simulink model "AreaCoverageTestHarness"  (R2016a)
settings: Solver=FixedStepDiscrete  StartTime=0.0  StopTime=6000  FixedStep=0.005  RelTol=1e-3
values from neighbouring files (symbols this model uses):
  BLOCK_SIZE = CAL_BLOCK_SIZE    [AreaCoverageCalib.m]    (also in room_V1.m = 20; room_V3.m = 20)
  EAST = 0    [AreaCoverageCalib.m]
  ERRVAL = 5    [AreaCoverageCalib.m]
  initXSim = 35    [AreaCoverageCalib.m]
  initYSim = 50    [AreaCoverageCalib.m]
  MAX_SPEED = 1000    [AreaCoverageCalib.m]
  MOTOR_HIGH = CAL_MOTOR_HIGH    [AreaCoverageCalib.m]
  MOTOR_LOW = CAL_MOTOR_LOW    [AreaCoverageCalib.m]
  NORTH = 270    [AreaCoverageCalib.m]
  PLOT_SAMPLE = 10    [AreaCoverageCalib.m]
  ROB_LENG = CAL_ROBO_LENG    [AreaCoverageCalib.m]
  ROB_WHEEL_R = .15    (= 0.15)    [AreaCoverageCalib.m]
  room = uint8(ones(side_size , side_size)*255)    [room_V1.m]    (also in room_V3.m)
  ROOM_SIDE_SIZE = CAL_ROOM_SIDE_SIZE    [AreaCoverageCalib.m]    (also in room_V1.m = 20; room_V3.m = 20)
  SAMPLE_TIME = 0.001    [AreaCoverageCalib.m]
  SOUTH = 90    [AreaCoverageCalib.m]
  STEP_SIZE = 5    [AreaCoverageCalib.m]
  WEST = 180    [AreaCoverageCalib.m]
undefined symbols (not defined in the file or in its folder): ROBO_LENG, sigbuilder_block
libraries: simulink x4
(part 2 of 2)

== stateflow chart AreaCoverageTestHarness/Robot/RoomFilterSystem/Chart ==
  state hitFlag = westHitCheck(c_x, c_y) [function]
    (default) -> (junction 455) : {xCount = relSizeUnit;
        | yCount = 1;}
    (junction 455) -> (junction 452) [order 1] : [room[c_x - xCount][c_y - yCount] == 0]// fourth quadrant up left
    (junction 456) -> (junction 455) : {
        | xCount--;
        | yCount++;
        | }
    (junction 455) -> (junction 454) [order 2]
    (junction 452) -> (junction 451)
    (junction 454) -> (junction 456) [order 1] : [xCount > 0]
    (junction 454) -> (junction 450) [order 2] : {xCount = relSizeUnit;}
    (junction 450) -> (junction 451) [order 1] : [room[c_x - xCount][c_y] == 0]// West
    (junction 450) -> (junction 448) [order 2] : {xCount = relSizeUnit;
        | yCount = 1;}
    (junction 451) -> (junction 447)
    (junction 448) -> (junction 447) [order 1] : [room[c_x - xCount][c_y + yCount] == 0]// third quadrant down left
    (junction 446) -> (junction 448) : {
        | xCount--;
        | yCount++;
        | }
    (junction 448) -> (junction 453) [order 2]
    (junction 447) -> (junction 443) : {hitFlag = true;}
    (junction 453) -> (junction 446) [order 1] : [xCount > 0]
    (junction 453) -> (junction 445) [order 2] : {hitFlag = false;}
    (junction 443) -> (junction 445)
  state hitFlag = southHitCheck(c_x, c_y) [function]
    (default) -> (junction 387) : {
        | xCount = relSizeUnit;
        | yCount = 1;
        | }
    (junction 387) -> (junction 384) [order 1] : [room[c_x - xCount][c_y + yCount] == 0]// third quadrant down left
    (junction 388) -> (junction 387) : {
        | xCount--;
        | yCount++;
        | }
    (junction 387) -> (junction 386) [order 2]
    (junction 384) -> (junction 383)
    (junction 386) -> (junction 388) [order 1] : [xCount > 0]
    (junction 386) -> (junction 382) [order 2] : {yCount = relSizeUnit;}
    (junction 382) -> (junction 383) [order 1] : [room[c_x][c_y + yCount] == 0]// south
    (junction 382) -> (junction 380) [order 2] : {xCount = relSizeUnit;
        | yCount = 1;}
    (junction 383) -> (junction 379)
    (junction 380) -> (junction 379) [order 1] : [room[c_x + xCount][c_y + yCount] == 0]// second quadrant down right
    (junction 378) -> (junction 380) : {
        | xCount--;
        | yCount++;
        | }
    (junction 380) -> (junction 385) [order 2]
    (junction 379) -> (junction 375) : {hitFlag = true;}
    (junction 385) -> (junction 378) [order 1] : [xCount > 0]
    (junction 385) -> (junction 377) [order 2] : {hitFlag = false;}
    (junction 375) -> (junction 377)
  state hitFlag = eastHitCheck(c_x, c_y) [function]
    (default) -> (junction 421) : {xCount = relSizeUnit;
        | yCount = 1;}
    (junction 421) -> (junction 418) [order 1] : [room[c_x + xCount][c_y + yCount] == 0]// second quadrant down right
    (junction 422) -> (junction 421) : {
        | xCount--;
        | yCount++;
        | }
    (junction 421) -> (junction 420) [order 2]
    (junction 418) -> (junction 417)
    (junction 420) -> (junction 422) [order 1] : [xCount > 0]
    (junction 420) -> (junction 416) [order 2] : {xCount = relSizeUnit;}
    (junction 416) -> (junction 417) [order 1] : [room[c_x + xCount][c_y] == 0]// East
    (junction 416) -> (junction 414) [order 2] : {xCount = 1;
        | yCount = relSizeUnit;}
    (junction 417) -> (junction 413)
    (junction 414) -> (junction 413) [order 1] : [room[c_x + xCount][c_y - yCount] == 0]// first quadrant up right
    (junction 412) -> (junction 414) : {
        | xCount++;
        | yCount--;
        | }
    (junction 414) -> (junction 419) [order 2]
    (junction 413) -> (junction 409) : {hitFlag = true;}
    (junction 419) -> (junction 412) [order 1] : [yCount > 0]
    (junction 419) -> (junction 411) [order 2] : {hitFlag = false;}
    (junction 409) -> (junction 411)
  state hitFlag = northHitCheck(c_x, c_y) [function]
    (default) -> (junction 337) : {xCount = relSizeUnit;
        | yCount = 1;}
    (junction 337) -> (junction 335) [order 1] : [room[c_x - xCount][c_y - yCount] == 0]// fourth quadrant up left
    (junction 336) -> (junction 337) : {
        | xCount--;
        | yCount++;
        | }
    (junction 337) -> (junction 332) [order 2]
    (junction 335) -> (junction 345)
    (junction 332) -> (junction 336) [order 1] : [xCount > 0]
    (junction 332) -> (junction 344) [order 2] : {yCount = relSizeUnit;}
    (junction 344) -> (junction 345) [order 1] : [room[c_x][c_y - yCount] == 0]// north
    (junction 344) -> (junction 355) [order 2] : {xCount = 1;
        | yCount = relSizeUnit;}
    (junction 345) -> (junction 353)
    (junction 355) -> (junction 353) [order 1] : [room[c_x + xCount][c_y - yCount] == 0]// first quadrant up right
    (junction 354) -> (junction 355) : {
        | xCount++;
        | yCount--;
        | }
    (junction 355) -> (junction 350) [order 2]
    (junction 353) -> (junction 359) : {hitFlag = true;}
    (junction 350) -> (junction 354) [order 1] : [yCount > 0]
    (junction 350) -> (junction 360) [order 2] : {hitFlag = false;}
    (junction 359) -> (junction 360)
  state noHit
    entry:
    hit_BOOL = false;
  state HitCalcHeading
    entry:
    hit_BOOL = true;
    during:
    c_x = x_raw - 1;
    c_y = y_raw - 1;
    (default) -> (junction 163)
    (junction 163) -> (junction 164) [order 1] : [(theta <= 270+ERRVAL) && (theta >= 270 - ERRVAL)]//NORTH
    (junction 163) -> (junction 165) [order 2]
    (junction 164) -> (junction 178) : {heading = NORTH;}
    (junction 165) -> (junction 166) [order 1] : [(theta <= 90+ERRVAL) && (theta >= 90-ERRVAL)]//SOUTH
    (junction 165) -> (junction 167) [order 2]
    (junction 166) -> (junction 177) : {heading = SOUTH;}
    (junction 167) -> (junction 168) [order 1] : [(theta <= 0+ERRVAL) || (theta >= 360-ERRVAL)]//EAST
    (junction 167) -> (junction 169) [order 2]
    (junction 168) -> (junction 176) : {heading = EAST;}
    (junction 169) -> (junction 170) [order 1] : [(theta <= 180+ERRVAL) && (theta >= 180-ERRVAL)]//WEST
    (junction 169) -> (junction 171) [order 2] : {heading = NONE;}
    (junction 170) -> (junction 175) : {heading = WEST;}
    (junction 171) -> (junction 172) [order 2] : [Vr == Vl]
    (junction 172) -> (junction 174) : {wrongHeading_BOOL = true;}
    (junction 171) -> (junction 173) [order 1]
    (junction 174) -> (junction 173)
    (junction 175) -> (junction 174) : {wrongHeading_BOOL = false;}
    (junction 176) -> (junction 175)
    (junction 177) -> (junction 176)
    (junction 178) -> (junction 177)
    (junction 173) -> (junction 179)
  state CalcHeading
    entry:
    y_out = y_raw ;
    x_out = x_raw ;
    c_x = x_raw - 1; // X and Y in C arrays are flipped
    c_y = y_raw - 1;
    during:
    y_out = y_raw;
    x_out = x_raw ;
    c_x = x_raw - 1; // X and Y in C arrays are flipped
    c_y = y_raw - 1;
    (default) -> (junction 66)
    (junction 66) -> (junction 67) [order 1] : [(theta <= 270+ERRVAL) && (theta >= 270 - ERRVAL)]//NORTH
    (junction 66) -> (junction 68) [order 2]
    (junction 67) -> (junction 75) : {heading = NORTH;}
    (junction 68) -> (junction 69) [order 1] : [(theta <= 90+ERRVAL) && (theta >= 90-ERRVAL)]//SOUTH
    (junction 68) -> (junction 70) [order 2]
    (junction 69) -> (junction 74) : {heading = SOUTH;}
    (junction 70) -> (junction 71) [order 1] : [(theta <= 0+ERRVAL) || (theta >= 360-ERRVAL)]//EAST
    (junction 70) -> (junction 80) [order 2]
    (junction 71) -> (junction 73) : {heading = EAST;}
    (junction 80) -> (junction 79) [order 1] : [(theta <= 180+ERRVAL) && (theta >= 180-ERRVAL)]//WEST
    (junction 80) -> (junction 128) [order 2] : {heading = NONE;}
    (junction 79) -> (junction 77) : {heading = WEST;}
    (junction 128) -> (junction 125) [order 2] : [Vr == Vl]
    (junction 125) -> (junction 126) : {wrongHeading_BOOL = true;}
    (junction 128) -> (junction 72) [order 1]
    (junction 126) -> (junction 72)
    (junction 77) -> (junction 126) : {wrongHeading_BOOL = false;}
    (junction 73) -> (junction 77)
    (junction 74) -> (junction 73)
    (junction 75) -> (junction 74)
    (junction 72) -> (junction 76)
  (default) -> noHit
  (junction 157) -> (junction 147) [order 3] : [(heading == NORTH) ...
      | && ((c_y - 1) >= 0)...
      | &&((c_x) >= 0)]
  (junction 147) -> noHit : [room[c_x][c_y - 1] == 255]
  (junction 146) -> noHit : [room[c_x + 1][c_y] == 255]
  (junction 157) -> (junction 146) [order 2] : [(heading == EAST) ...
      | && ((c_x) <= 150 - 1)...
      | && ((c_y) >= 0)]
  (junction 92) -> HitCalcHeading : [northHitCheck(c_x, c_y)]
  (junction 109) -> (junction 92) [order 2] : [(heading == NORTH) ...
      | && ((c_y - 1) >= 0)...
      | &&((c_x) >= 0)]
  CalcHeading -> CalcHeading [order 3] : [hasChanged(theta)]
  HitCalcHeading -> (junction 157) [order 1] : [(Vr > 0) && (Vl > 0)]//FORWARD
  (junction 157) -> (junction 148) [order 4] : [(heading == SOUTH) ...
      | && ((c_y + 1) <= 150 - 1)...
      | && ((c_x) >= 0)]
  (junction 157) -> (junction 145) [order 1] : [(heading == WEST) ...
      | && ((c_x - 1) >= 0)...
      | && ((c_y) >= 0)]
  (junction 148) -> noHit : [room[c_x][c_y + 1] == 255]
  (junction 97) -> HitCalcHeading : [eastHitCheck(c_x, c_y)]
  (junction 109) -> (junction 97) [order 4] : [(heading == EAST) ...
      | && ((c_x) <= 150 - 1)...
      | && ((c_y) >= 0)]
  CalcHeading -> (junction 109) [order 1] : [(Vr > 0) && (Vl > 0)]//FORWARD
  (junction 109) -> (junction 100) [order 1] : [(heading == SOUTH) ...
      | && ((c_y + 1) <= 150 - 1)...
      | && ((c_x) >= 0)]
  (junction 109) -> (junction 103) [order 3] : [(heading == WEST) ...
      | && ((c_x - 1) >= 0)...
      | && ((c_y) >= 0)]
  (junction 145) -> noHit : [room[c_x - 1][c_y] == 255]
  (junction 100) -> HitCalcHeading : [southHitCheck(c_x, c_y)]
  HitCalcHeading -> noHit [order 4]
  (junction 103) -> HitCalcHeading : [westHitCheck(c_x, c_y)]
  (junction 135) -> noHit : [room[c_y + 1][c_x] == 255]
  (junction 160) -> (junction 135) [order 1] : [(heading == NORTH) ...
      | && ((c_y + 1) <= 150 - 1)...
      | && ((c_x) >= 0)]
  (junction 111) -> (junction 113) [order 1] : [(heading == NORTH) ...
      | && ((c_y + 1) <= 150 - 1)...
      | && ((c_x) >= 0)]
  (junction 113) -> HitCalcHeading : [room[c_y + 1][c_x] == 0]
  CalcHeading -> (junction 111) [order 2] : [(Vr < 0) && (Vl < 0)]//BACKWARD
  (junction 111) -> (junction 114) [order 2] : [(heading == EAST) ...
      | && ((c_x - 1) >= 0)...
      | && ((c_y) >= 0)]
  (junction 111) -> (junction 115) [order 3] : [(heading == SOUTH) ...
      | && ((c_y - 1) >= 0)...
      | && ((c_x) >=0)]
  (junction 111) -> (junction 116) [order 4] : [(heading == WEST) ...
      | && ((c_x + 1) <= (150-1))...
      | && ((c_y) >= 0)]
  (junction 114) -> HitCalcHeading : [room[c_y][c_x - 1] == 0]
  HitCalcHeading -> (junction 160) [order 2] : [(Vr < 0) && (Vl < 0)]//BACKWARD
  (junction 160) -> (junction 138) [order 2] : [(heading == EAST) ...
      | && ((c_x - 1) >= 0)...
      | && ((c_y) >= 0)]
  (junction 138) -> noHit : [room[c_y][c_x - 1] == 255]
  (junction 160) -> (junction 134) [order 3] : [(heading == SOUTH) ...
      | && ((c_y - 1) >= 0)...
      | && ((c_x) >=0)]
  (junction 160) -> (junction 136) [order 4] : [(heading == WEST) ...
      | && ((c_x + 1) <= (150-1))...
      | && ((c_y) >= 0)]
  noHit -> CalcHeading
  (junction 115) -> HitCalcHeading : [(room[c_y - 1][c_x] == 0)]
  (junction 134) -> noHit : [room[c_y - 1][c_x] == 255]
  (junction 116) -> HitCalcHeading : [room[c_y][c_x + 1] == 0]
  HitCalcHeading -> HitCalcHeading [order 3] : [hasChanged(theta)]
  (junction 136) -> noHit : [room[c_y][c_x + 1] == 255]
  data: c_x function_input double; c_y function_input double; hitFlag function_output boolean; i temporary int8; c_x function_input double; c_y function_input double; hitFlag function_output boolean; i temporary int8; c_x function_input double; c_y function_input double; hitFlag function_output boolean; i temporary int8; c_x function_input double; c_y function_input double; hitFlag function_output boolean; i temporary int8; x_raw input; y_raw input; room input size=[ROOM_SIDE_SIZE*BLOCK_SIZE/4 ROOM_SIDE_SIZE*BLOCK_SIZE/4]; y_out output int32; x_out output int32; y_temp local int32; x_temp local int32; hit_BOOL output boolean; theta input; ERRVAL input; NORTH input; SOUTH input; EAST input; WEST input; NONE input; heading local int16; Vr input; Vl input; wrongHeading_BOOL output boolean; c_x local double; c_y local double; relSizeUnit constant double =uint8(ROB_LENG/STEP_SIZE/2); xCount local double; yCount local double

== stateflow chart AreaCoverageTestHarness/Robot/RoomFilterSystem/StepCalc/Chart ==
  state inStep
    entry:
    temp = 0;
    state wait
    (default) -> wait
    (junction 7) -> wait : [oldPos < pos]/temp++;
    wait -> (junction 5) [order 1] : [hasChanged(pos)]
    (junction 5) -> wait : [oldPos > pos]/temp--;
    wait -> (junction 7) [order 2] : [hasChanged(pos)]
  state IncrementStep
    entry:
    step++;
  state Start
    entry:
    step = pos;
  state decrementStep
    step--;
  (default) -> Start
  Start -> inStep
  inStep -> IncrementStep [order 1] : [temp >= STEP_SIZE]
  IncrementStep -> inStep
  decrementStep -> inStep
  inStep -> decrementStep [order 2] : [temp <= -STEP_SIZE]
  data: pos input; oldPos input; step output int32; temp local int8; STEP_SIZE input int8

== stateflow chart AreaCoverageTestHarness/Robot/OrientationCalculator/VelocityCalculator/Chart2 ==
  (default) -> (junction 96)
  (junction 96) -> (junction 110) [order 1] : [(!LeftMotorPosPin_BOOL && !LeftMotorNegPin_BOOL && !RightMotorPosPin_BOOL && !RightMotorNegPin_BOOL)...
      | || (LeftMotorPosPin_BOOL && LeftMotorNegPin_BOOL && !RightMotorPosPin_BOOL && !RightMotorNegPin_BOOL)...
      | || (!LeftMotorPosPin_BOOL && !LeftMotorNegPin_BOOL && RightMotorPosPin_BOOL && RightMotorNegPin_BOOL)...
      | || (LeftMotorPosPin_BOOL && LeftMotorNegPin_BOOL && RightMotorPosPin_BOOL && RightMotorNegPin_BOOL)]
  (junction 110) -> (junction 118) : {Vr  = 0;
      | Vl = 0;}
  (junction 96) -> (junction 100) [order 2]
  (junction 100) -> (junction 97) [order 1] : [(!LeftMotorPosPin_BOOL && !LeftMotorNegPin_BOOL && RightMotorPosPin_BOOL && !RightMotorNegPin_BOOL)...
      | || (!LeftMotorPosPin_BOOL && LeftMotorNegPin_BOOL && RightMotorPosPin_BOOL && RightMotorNegPin_BOOL)...
      | || (LeftMotorPosPin_BOOL && LeftMotorNegPin_BOOL && RightMotorPosPin_BOOL && !RightMotorNegPin_BOOL)...
      | || (!LeftMotorPosPin_BOOL && LeftMotorNegPin_BOOL && !RightMotorPosPin_BOOL && !RightMotorNegPin_BOOL)]
  (junction 97) -> (junction 122) : {Vr = MAX_SPEED;
      | Vl = 0;}
  (junction 100) -> (junction 99) [order 2]
  (junction 99) -> (junction 98) [order 1] : [(!LeftMotorPosPin_BOOL && !LeftMotorNegPin_BOOL && !RightMotorPosPin_BOOL && RightMotorNegPin_BOOL)...
      | || (LeftMotorPosPin_BOOL && !LeftMotorNegPin_BOOL && !RightMotorPosPin_BOOL && !RightMotorNegPin_BOOL)...
      | || (LeftMotorPosPin_BOOL && !LeftMotorNegPin_BOOL && RightMotorPosPin_BOOL && RightMotorNegPin_BOOL)...
      | || (LeftMotorPosPin_BOOL && LeftMotorNegPin_BOOL && !RightMotorPosPin_BOOL && RightMotorNegPin_BOOL)]
  (junction 98) -> (junction 86) : {Vr = 0;
      | Vl = MAX_SPEED;}
  (junction 99) -> (junction 87) [order 2]
  (junction 87) -> (junction 101) [order 1] : [(!LeftMotorPosPin_BOOL && LeftMotorNegPin_BOOL && RightMotorPosPin_BOOL && !RightMotorNegPin_BOOL)]
  (junction 87) -> (junction 102) [order 2]
  (junction 101) -> (junction 130) : {Vr = MAX_SPEED;
      | Vl = -MAX_SPEED;}
  (junction 102) -> (junction 104) [order 1] : [(LeftMotorPosPin_BOOL && !LeftMotorNegPin_BOOL && !RightMotorPosPin_BOOL && RightMotorNegPin_BOOL)]
  (junction 102) -> (junction 133) [order 2]
  (junction 104) -> (junction 88) : {Vr = -MAX_SPEED;
      | Vl = MAX_SPEED;}
  (junction 133) -> (junction 105) [order 1] : [(LeftMotorPosPin_BOOL && !LeftMotorNegPin_BOOL && RightMotorPosPin_BOOL && !RightMotorNegPin_BOOL)]
  (junction 133) -> (junction 90) [order 2]
  (junction 105) -> (junction 89) : {Vr = MAX_SPEED;
      | Vl = MAX_SPEED;}
  (junction 90) -> (junction 94) [order 1] : [(!LeftMotorPosPin_BOOL && LeftMotorNegPin_BOOL && !RightMotorPosPin_BOOL && RightMotorNegPin_BOOL)]
  (junction 90) -> (junction 91) [order 2]
  (junction 94) -> (junction 127) : {Vr = -MAX_SPEED;
      | Vl = -MAX_SPEED;}
  (junction 127) -> (junction 91)
  (junction 89) -> (junction 127)
  (junction 88) -> (junction 89)
  (junction 130) -> (junction 88)
  (junction 86) -> (junction 130)
  (junction 122) -> (junction 86)
  (junction 118) -> (junction 122)
  (junction 91) -> (junction 119)
  data: LeftMotorPosPin_BOOL input; LeftMotorNegPin_BOOL input; RightMotorPosPin_BOOL input; RightMotorNegPin_BOOL input; Vr output int16 =0; Vl output int16 =0; MAX_SPEED input int16

== stateflow chart AreaCoverageTestHarness/Robot/RoomFilterSystem/StepCalc1/Chart ==
  state inStep
    entry:
    temp = 0;
    state wait
    (default) -> wait
    (junction 7) -> wait : [oldPos < pos]/temp++;
    wait -> (junction 5) [order 1] : [hasChanged(pos)]
    (junction 5) -> wait : [oldPos > pos]/temp--;
    wait -> (junction 7) [order 2] : [hasChanged(pos)]
  state IncrementStep
    entry:
    step++;
  state Start
    entry:
    step = pos;
  state decrementStep
    step--;
  (default) -> Start
  Start -> inStep
  inStep -> IncrementStep [order 1] : [temp >= STEP_SIZE]
  IncrementStep -> inStep
  decrementStep -> inStep
  inStep -> decrementStep [order 2] : [temp <= -STEP_SIZE]
  data: pos input; oldPos input; step output int32; temp local int8; STEP_SIZE input int8

== stateflow chart AreaCoverageTestHarness/Robot/ULS_Calc/ULS_Calculation ==
  state WestCalc
    entry:
    leftCounter = y - 1;
    rightCounter = y - 1;
    ULSL = 0;
    ULSR = 0;
    startLeft = true;
    startRight = true;
    state ULSL [parallel]
      settings: executionOrder=2
      (default) -> (junction 333)
      (junction 333) -> (junction 344) [order 1] : [leftCounter + 1 <= roomSize]
      (junction 336) -> (junction 333) : {ULSL++;}
      (junction 333) -> (junction 334) [order 2]
      (junction 344) -> (junction 335) : {leftCounter++;}
      (junction 334) -> (junction 336) [order 1] : [room[x-1][leftCounter] == 255]
      (junction 335) -> (junction 334)
      (junction 334) -> (junction 341) [order 2] : //if room[rightCounter][y - 1] == 0
    state ULSR [parallel]
      settings: executionOrder=1
      (default) -> (junction 347)
      (junction 347) -> (junction 358) [order 1] : [rightCounter - 1 >= 0]
      (junction 350) -> (junction 347) : {ULSR++;}
      (junction 347) -> (junction 348) [order 2]
      (junction 358) -> (junction 349) : {rightCounter--;}
      (junction 348) -> (junction 350) [order 1] : [room[x-1][rightCounter] == 255]
      (junction 349) -> (junction 348)
      (junction 348) -> (junction 355) [order 2] : //if room[rightCounter][y - 1] == 0
  state NorthCalc
    entry:
    leftCounter = x-1;
    rightCounter = x-1;
    ULSL = 0;
    ULSR = 0;
    startLeft = true;
    startRight = true;
    state ULSL [parallel]
      settings: executionOrder=1
      (default) -> (junction 232)
      (junction 232) -> (junction 236) [order 1] : [leftCounter - 1 >= 0]
      (junction 234) -> (junction 232) : {ULSL++;}
      (junction 232) -> (junction 193) [order 2]
      (junction 236) -> (junction 237) : {leftCounter--;}
      (junction 193) -> (junction 234) [order 1] : [room[leftCounter][y-1] == 255]
      (junction 237) -> (junction 193)
      (junction 193) -> (junction 233) [order 2]
    state ULSR [parallel]
      settings: executionOrder=2
      (default) -> (junction 258)
      (junction 258) -> (junction 250) [order 1] : [rightCounter + 1 <= roomSize]
      (junction 251) -> (junction 258) : {ULSR++;}
      (junction 258) -> (junction 253) [order 2]
      (junction 250) -> (junction 271) : {rightCounter++;}
      (junction 253) -> (junction 251) [order 1] : [room[rightCounter][y - 1] == 255]
      (junction 271) -> (junction 253)
      (junction 253) -> (junction 272) [order 2] : //if room[rightCounter][y - 1] == 0
  state CalcHeading
    (default) -> (junction 2)
    (junction 2) -> (junction 3) [order 1] : [(theta <= 270+ERRVAL) && (theta >= 270 - ERRVAL)]//NORTH
    (junction 2) -> (junction 4) [order 2]
    (junction 3) -> (junction 17) : {heading = NORTH;}
    (junction 4) -> (junction 5) [order 1] : [(theta <= 90+ERRVAL) && (theta >= 90-ERRVAL)]//SOUTH
    (junction 4) -> (junction 6) [order 2]
    (junction 5) -> (junction 16) : {heading = SOUTH;}
    (junction 6) -> (junction 7) [order 1] : [(theta <= 0+ERRVAL) || (theta >= 360-ERRVAL)]//EAST
    (junction 6) -> (junction 8) [order 2]
    (junction 7) -> (junction 15) : {heading = EAST;}
    (junction 8) -> (junction 9) [order 1] : [(theta <= 180+ERRVAL) && (theta >= 180-ERRVAL)]//WEST
    (junction 8) -> (junction 10) [order 2] : {heading = NONE;}
    (junction 9) -> (junction 14) : {heading = WEST;}
    (junction 10) -> (junction 11) [order 1] : [Vr == Vl]
    (junction 11) -> (junction 13) : {wrongHeading_BOOL = true;}
    (junction 10) -> (junction 12) [order 2]
    (junction 13) -> (junction 12)
    (junction 14) -> (junction 13) : {wrongHeading_BOOL = false;}
    (junction 15) -> (junction 14)
    (junction 16) -> (junction 15)
    (junction 17) -> (junction 16)
    (junction 12) -> (junction 18)
  state EastCalc
    entry:
    leftCounter = y-1;
    rightCounter = y-1;
    ULSL = 0;
    ULSR = 0;
    startLeft = true;
    startRight = true;
    state ULSL [parallel]
      settings: executionOrder=2
      (default) -> (junction 305)
      (junction 305) -> (junction 316) [order 1] : [leftCounter - 1 >= 0]
      (junction 308) -> (junction 305) : {ULSL++;}
      (junction 305) -> (junction 306) [order 2]
      (junction 316) -> (junction 307) : {leftCounter--;}
      (junction 306) -> (junction 308) [order 1] : [room[x-1][leftCounter] == 255]
      (junction 307) -> (junction 306)
      (junction 306) -> (junction 313) [order 2] : //if room[rightCounter][y - 1] == 0
    state ULSR [parallel]
      settings: executionOrder=1
      (default) -> (junction 319)
      (junction 319) -> (junction 330) [order 1] : [rightCounter + 1 <= roomSize]
      (junction 322) -> (junction 319) : {ULSR++;}
      (junction 319) -> (junction 320) [order 2]
      (junction 330) -> (junction 321) : {rightCounter++;}
      (junction 320) -> (junction 322) [order 1] : [room[x-1][rightCounter] == 255]
      (junction 321) -> (junction 320)
      (junction 320) -> (junction 327) [order 2] : //if room[rightCounter][y - 1] == 0
  state SouthCalc
    entry:
    leftCounter = x-1;
    rightCounter = x-1;
    ULSL = 0;
    ULSR = 0;
    startLeft = true;
    startRight = true;
    state ULSL [parallel]
      settings: executionOrder=1
      (default) -> (junction 278)
      (junction 278) -> (junction 288) [order 1] : [leftCounter + 1 <= roomSize]
      (junction 279) -> (junction 278) : {ULSL++;}
      (junction 278) -> (junction 286) [order 2]
      (junction 288) -> (junction 281) : {leftCounter++;}
      (junction 286) -> (junction 279) [order 1] : [room[leftCounter][y-1] == 255]
      (junction 281) -> (junction 286)
      (junction 286) -> (junction 283) [order 2] : //if room[leftCounter][y - 1] == 0
    state ULSR [parallel]
      settings: executionOrder=2
      (default) -> (junction 292)
      (junction 292) -> (junction 302) [order 1] : [rightCounter - 1 >= 0]
      (junction 293) -> (junction 292) : {ULSR++;}
      (junction 292) -> (junction 300) [order 2]
      (junction 302) -> (junction 295) : {rightCounter--;}
      (junction 300) -> (junction 293) [order 1] : [room[rightCounter][y - 1] == 255]
      (junction 295) -> (junction 300)
      (junction 300) -> (junction 297) [order 2] : //if room[rightCounter][y - 1] == 0
  (default) -> CalcHeading
  CalcHeading -> WestCalc [order 1] : [(heading == WEST) ...
      | && (hasChanged(heading)...
      | || hasChanged(x))]
      | /readingReady = false;
  CalcHeading -> NorthCalc [order 4] : [(heading == NORTH) ...
      | && (hasChanged(heading)...
      | || hasChanged(y))]
      | /readingReady = false;
  (junction 154) -> CalcHeading : [(room[x-1][rightCounter] == 0)...
      |  &&(room[x-1][leftCounter] == 0)]
      | /readingReady = true;
  WestCalc -> (junction 154) : [x-1 >= 0]
  EastCalc -> (junction 154) : [x-1 >= 0]
  NorthCalc -> (junction 117) : [y-1 >= 0]
  (junction 117) -> CalcHeading : [(room[rightCounter][y-1] == 0)...
      |  &&(room[leftCounter][y-1] == 0)]
      | /readingReady = true;
  SouthCalc -> (junction 117) : [y-1 >= 0]
  CalcHeading -> EastCalc [order 2] : [(heading == EAST) ...
      | && (hasChanged(heading)...
      | || hasChanged(x))]
      | /readingReady = false;
  CalcHeading -> SouthCalc [order 3] : [(heading == SOUTH) ...
      | && (hasChanged(heading)...
      | || hasChanged(y))]
      | /readingReady = false;
  CalcHeading -> CalcHeading [order 5] : [hasChanged(theta)]
  data: ERRVAL input; NORTH input; SOUTH input; EAST input; WEST input; NONE input; room input size=[ROOM_SIDE_SIZE*BLOCK_SIZE/4 ROOM_SIDE_SIZE*BLOCK_SIZE/4]; heading local int16; theta input; Vl input; Vr input; roomSize input; x input; y input; wrongHeading_BOOL output double; ULSL output double; ULSR output double; leftCounter local double; rightCounter local double; startLeft local boolean; startRight local boolean; readingReady output boolean

== matlab function AreaCoverageTestHarness/Robot/DetailedMap/MATLAB Function ==
  data: room input; X input; Y input; Theta input; ROOM_SIDE_SIZE parameter; clock input; BLOCK_SIZE parameter
function PlotterFunc(room, X, Y, Theta, ROOM_SIDE_SIZE, clock, BLOCK_SIZE)

persistent init;
persistent fig;

if isempty(fig)
    fig = figure;
end

if isempty(init)
    init = 0;
    %room = uint8(room');
    hold off;
    clf
    empty = 255;
    busy = 0;
    hold on
    offset = 0;
    for i = 1:length(room(1, :))
        for j = 1:length(room(:, 1))
            if room(i, j) == empty
%                 plot(i - offset, j - offset, '*b');
            else if room(i,j) == busy
                    plot(i - offset, j - offset, '.r');
                else 
                    plot(i - offset, j - offset, 'x');
                end
            end
        end
    end
    axis ij
end


delta = clock - init;
if(delta) >= 0.5
%     figure(fig);
    init = clock;
    Xplot = double(X);
    Yplot = double(Y);
        if clock
%             hold on
            lineLength = double(BLOCK_SIZE*0.25);
            opleft = double(sind(Theta+90) * (lineLength/2));
            adjleft = double(cosd(Theta+90) * (lineLength/2));
            yend = double(Yplot) + opleft;
            xend = double(Xplot) + adjleft;
            start = [double(Xplot) xend];
            finish = [double(Yplot) yend];

            opright = double(sind(Theta-90) * (lineLength/2));
            adjright = double(cosd(Theta-90) * (lineLength/2));

            plot(double(Xplot), double(Yplot), 'r*', 'MarkerSize', 10);
            hold on

            plot(start, finish, 'g', 'LineWidth', 3)
            plot(xend, yend, 'bx')
            yend = double(Yplot) + opright;
            xend = double(Xplot) + adjright;
            start = [double(Xplot) xend];
            finish = [double(Yplot) yend];
            plot(start, finish, 'g','LineWidth', 3)
            plot(xend, yend, 'bx')
%             hold off
%             xlim([-1*((ROOM_SIDE_SIZE * BLOCK_SIZE)/2) - 50 (ROOM_SIDE_SIZE * BLOCK_SIZE)/2 + 50]);
%             ylim([-1*((ROOM_SIDE_SIZE * BLOCK_SIZE)/2) - 50 (ROOM_SIDE_SIZE * BLOCK_SIZE)/2 + 50]);
            xlim([0 100]);
            ylim([0 100]);
            grid on
            grid minor
%                 hold off;

    %         axis ij
        end
end

== stateflow chart AreaCoverageTestHarness/Robot/PlotSampler ==
  (default) -> (junction 1)
  (junction 1) -> (junction 3) : {counter = counter + 1;...
      | Event_BOOL = false;}
  (junction 3) -> (junction 5) [order 1] : [counter >= PLOT_SAMPLE]
  (junction 3) -> (junction 9) [order 2] : /{Event_BOOL = false;}
  (junction 5) -> (junction 7) : {counter = 0;...
      | Event_BOOL = true;}
  (junction 7) -> (junction 9)
  data: counter local uint8; Event_BOOL output boolean; PLOT_SAMPLE input

== matlab function AreaCoverageTestHarness/Robot/DetailedMap/createMap/RoomV3/Room_V3 ==
  data: roomOut output size=[ROOM_SIDE_SIZE*BLOCK_SIZE/4 ROOM_SIDE_SIZE*BLOCK_SIZE/4] [0..255]; ROOM_SIDE_SIZE parameter; BLOCK_SIZE parameter
function roomOut = fcn(ROOM_SIDE_SIZE, BLOCK_SIZE)

persistent flag;
persistent room;
   side_size = ROOM_SIDE_SIZE * (BLOCK_SIZE/4);

if isempty(flag)
    flag = false;
    room = uint8(ones(side_size , side_size)*255);
end

if flag == false
   flag = true;
%     room = uint8(ones(ROOM_SIDE_SIZE , ROOM_SIDE_SIZE)*255);

    %% Draw room Boarders
    for rowNum = 1:(side_size)
        for colNum = 1: side_size
            if (rowNum <= BLOCK_SIZE/4) || (rowNum >= (side_size - BLOCK_SIZE/4))...
                    || (colNum <= BLOCK_SIZE/4) || (colNum >= side_size - BLOCK_SIZE/4)
    %                 || (rowNum == 2) || (rowNum == roomSize - 1)...
    %                 || (colNum == 2) || (colNum == roomSize-1)
                room(rowNum, colNum) = 0;
            end
        end
    end

    %% Draw room Obsticals
    scale = 5;
    %% insert Table
    room((9*scale - scale/2) + 0.5:(11*scale + scale/2) + 0.5, (7*scale - scale/4) + 0.5:(13*scale + scale/4 )+ 0.5) = 0;
 
    %% insert chairs
    room((17*scale - scale/2) + 0.5:(19*scale + scale/2) + 0.5, (5*scale - (scale)/2) + 0.5:(8*scale + (scale)/2 )+ 0.5) = 0;

%     room((15.5*scale - scale/2) + 0.5:(17.5*scale + scale/2) + 0.5, (13*scale - (scale)/2) + 0.5:(16*scale + (scale)/2 )+ 0.5) = 0;

    room((9*scale - scale/2) + 0.5:(12*scale + scale/2) + 0.5, (17*scale - (scale)/2) + 0.5:(19*scale + (scale)/2 )+ 0.5) = 0;
    
    x = (14:0.1:16.5);
    y = (16:0.1:19);
    depth = 5;
    for j = 1:depth*scale
        for i = 1:length(x)
            room(uint8((x(i)*scale - scale/2) + 0.5), uint8((y(i)*scale - scale/2) + 0.5)) = 0;
        end
        x = x + 0.1;
        y = y - 0.1;
    end
    
    
    x = (2:0.1:5);
    y = (16.5:0.1:19.5);
    depth = 5;
    for j = 1:depth*scale
        for i = 1:length(x)
            room(uint8((x(i)*scale - scale/2) + 0.5), uint8((y(i)*scale - scale/2) + 0.5)) = 0;
        end
        x = x + 0.1;
        y = y - 0.1;
    end
    
    room((2*scale - scale/2) + 0.5:(4*scale + scale/2) + 0.5, (6*scale - (scale)/2) + 0.5:(13*scale + (scale)/2 )+ 0.5) = 0;
  
    roomOut = room;
else
    roomOut = room;
end

== stateflow chart AreaCoverageTestHarness/Robot/EncoderTicksGenerator/SquareWaveCreatorLeft ==
  state BulbOn
    state Off
      entry:
      counter = 0;
      encoderTicks_BOOL = false;
      du:
      counter++;
    state On
      entry:
      counter = 0;
      encoderTicks_BOOL = true;
      du:
      counter++;
    (default) -> Off
    On -> Off : [counter >= (spdGain)]/counter = 0;
    Off -> On : [counter >= (spdGain)]/counter = 0;
  state BulbOff
    entry:
    encoderTicks_BOOL = 0;
  (default) -> BulbOff
  BulbOff -> BulbOn : [ControlSignal_BOOL_in]
  BulbOn -> BulbOff : [!ControlSignal_BOOL_in]
  data: ControlSignal_BOOL_in input; encoderTicks_BOOL output boolean; counter local uint16; spdGain input

== matlab function AreaCoverageTestHarness/Robot/GridMap/MATLAB Function ==
  data: room input; X input; Y input; Theta input; ROOM_SIDE_SIZE parameter; clock input; BLOCK_SIZE parameter
function PlotterFunc(room, X, Y, Theta, ROOM_SIDE_SIZE, clock, BLOCK_SIZE)

persistent init;
persistent fig1;

if isempty(fig1)
    fig1 = figure;
end

if isempty(init)
    init = 0;
    %room = uint8(room');
    hold off;
    clf
    empty = 255;
    busy = 0;
    hold on
    offset = 0;
    for i = 1:length(room(1, :))
        for j = 1:length(room(:, 1))
            if room(i, j) == empty
                plot(i - offset, j - offset, '*b');
            else if room(i,j) == busy
                    plot(i - offset, j - offset, 'or');
                else 
                    plot(i - offset, j - offset, 'x');
                end
            end
        end
    end
    axis ij
end

delta = clock - init;
if(delta) >= 0.5
    figure(fig1);
    init = clock;
%     X = X - 1;
%     Y = Y - 1;
        if clock
            lineLength = double(BLOCK_SIZE*0.05);
            opleft = double(sind(Theta+90) * (lineLength/2));
            adjleft = double(cosd(Theta+90) * (lineLength/2));
            yend = double(Y) + opleft;
            xend = double(X) + adjleft;
            start = [double(X) xend];
            finish = [double(Y) yend];

            opright = double(sind(Theta-90) * (lineLength/2));
            adjright = double(cosd(Theta-90) * (lineLength/2));

            plot(double(X), double(Y), '*', 'MarkerSize', 10);
            hold on
            plot(start, finish, 'LineWidth', 3)
            plot(xend, yend, 'x')
            yend = double(Y) + opright;
            xend = double(X) + adjright;
            start = [double(X) xend];
            finish = [double(Y) yend];
            plot(start, finish, 'LineWidth', 3)
            plot(xend, yend, 'x')
%             hold off
            xlim([0 (ROOM_SIDE_SIZE)]);
            ylim([0 (ROOM_SIDE_SIZE)]);
            grid on
            grid minor
    %         axis ij
        end
end

== matlab function AreaCoverageTestHarness/Robot/createMap/MATLAB Function ==
  data: roomOut output size=[ROOM_SIDE_SIZE ROOM_SIDE_SIZE] [0..255]; ROOM_SIDE_SIZE parameter
function roomOut = fcn(  ROOM_SIDE_SIZE)

%persistent flag;
    room = uint8(ones(ROOM_SIDE_SIZE , ROOM_SIDE_SIZE)*255);
%if isempty(flag)
 %   flag = true;
%     room = uint8(ones(ROOM_SIDE_SIZE , ROOM_SIDE_SIZE)*255);

    %% Draw room Boarders
    for rowNum = 1:(ROOM_SIDE_SIZE)
        for colNum = 1: ROOM_SIDE_SIZE
            if (rowNum == 1) || (rowNum == ROOM_SIDE_SIZE)...
                    || (colNum == 1) || (colNum == ROOM_SIDE_SIZE)
    %                 || (rowNum == 2) || (rowNum == roomSize - 1)...
    %                 || (colNum == 2) || (colNum == roomSize-1)
                room(rowNum, colNum) = 0;
            end
        end
    end

    %% Draw room Obsticals

    %% insert Table
    room(4, 9) = 0;
    room(6, 9) = 0;
    room(4, 11) = 0;
    room(6, 11) = 0;

    %% insert box
    room(3:4, 4:5) = 0;

    %% insert soffa
    room(12:14, 8:13) = 0;

    %% insert LeglessTable
    room(7:11, 1:4) = 0;
    roomOut = room;
%else
  %  roomOut = room;
%end

== stateflow chart AreaCoverageTestHarness/Robot/ULS_Calc/ULS_Calculation1 ==
  state WestCalc
    entry:
    leftCounter = y - 1;
    rightCounter = y - 1;
    ULSL = 0;
    ULSR = 0;
    startLeft = true;
    startRight = true;
    state ULSL [parallel]
      settings: executionOrder=2
      (history)
      state ULSL_Calc
      state Hit
      WestCalc.ULSL.ULSL_Calc -> (junction 148) : [leftCounter + 1 <= roomSize]{leftCounter++;}
      (default) -> WestCalc.ULSL.ULSL_Calc
      (junction 148) -> WestCalc.ULSL.Hit [order 1] : [room[x-1][leftCounter] == 0]
          | /startLeft = false;
      (junction 148) -> WestCalc.ULSL.ULSL_Calc [order 2] : [room[x-1][leftCounter] == 255]
          | /ULSL++;
      WestCalc.ULSL.Hit -> WestCalc.ULSL.ULSL_Calc : [startLeft]
    state ULSR [parallel]
      settings: executionOrder=1
      (history)
      state ULSR_Calc1
      state Hit
      WestCalc.ULSR.ULSR_Calc1 -> (junction 147) : [rightCounter - 1 >= 0]{rightCounter--;}
      (default) -> WestCalc.ULSR.ULSR_Calc1
      (junction 147) -> WestCalc.ULSR.Hit [order 1] : [room[x-1][rightCounter] == 0]
          | /startRight = false;
      (junction 147) -> WestCalc.ULSR.ULSR_Calc1 [order 2] : [room[x-1][rightCounter] == 255]
          | /ULSR++;
      WestCalc.ULSR.Hit -> WestCalc.ULSR.ULSR_Calc1 : [startRight]
  state NorthCalc
    entry:
    leftCounter = x-1;
    rightCounter = x-1;
    ULSL = 0;
    ULSR = 0;
    startLeft = true;
    startRight = true;
    state ULSL [parallel]
      settings: executionOrder=2
      (history)
      state ULSL_Calc
      state Hit
      NorthCalc.ULSL.ULSL_Calc -> (junction 193) : [leftCounter - 1 >= 0]{leftCounter--;}
      (default) -> NorthCalc.ULSL.ULSL_Calc
      (junction 193) -> NorthCalc.ULSL.Hit [order 1] : [room[leftCounter][y-1]== 0]
          | /startLeft = false;
      (junction 193) -> NorthCalc.ULSL.ULSL_Calc [order 2] : [room[leftCounter][y-1] == 255]
          | /ULSL++;
      NorthCalc.ULSL.Hit -> NorthCalc.ULSL.ULSL_Calc : [startLeft]
    state ULSR [parallel]
      settings: executionOrder=1
      (history)
      state ULSR_Calc
      state Hit
      NorthCalc.ULSR.ULSR_Calc -> (junction 206) : [rightCounter + 1 <= roomSize]{rightCounter++;}
      (default) -> NorthCalc.ULSR.ULSR_Calc
      (junction 206) -> NorthCalc.ULSR.Hit [order 1] : [room[rightCounter][y - 1] == 0]
          | /startRight = false;
      (junction 206) -> NorthCalc.ULSR.ULSR_Calc [order 2] : [room[rightCounter][y - 1] == 255]
          | /ULSR++;
      NorthCalc.ULSR.Hit -> NorthCalc.ULSR.ULSR_Calc : [startRight]
  state CalcHeading
    (default) -> (junction 2)
    (junction 2) -> (junction 3) [order 1] : [(theta <= 270+ERRVAL) && (theta >= 270 - ERRVAL)]//NORTH
    (junction 2) -> (junction 4) [order 2]
    (junction 3) -> (junction 17) : {heading = NORTH;}
    (junction 4) -> (junction 5) [order 1] : [(theta <= 90+ERRVAL) && (theta >= 90-ERRVAL)]//SOUTH
    (junction 4) -> (junction 6) [order 2]
    (junction 5) -> (junction 16) : {heading = SOUTH;}
    (junction 6) -> (junction 7) [order 1] : [(theta <= 0+ERRVAL) || (theta >= 360-ERRVAL)]//EAST
    (junction 6) -> (junction 8) [order 2]
    (junction 7) -> (junction 15) : {heading = EAST;}
    (junction 8) -> (junction 9) [order 1] : [(theta <= 180+ERRVAL) && (theta >= 180-ERRVAL)]//WEST
    (junction 8) -> (junction 10) [order 2] : {heading = NONE;}
    (junction 9) -> (junction 14) : {heading = WEST;}
    (junction 10) -> (junction 11) [order 2] : [Vr == Vl]
    (junction 11) -> (junction 13) : {wrongHeading_BOOL = true;}
    (junction 10) -> (junction 12) [order 1]
    (junction 13) -> (junction 12)
    (junction 14) -> (junction 13) : {wrongHeading_BOOL = false;}
    (junction 15) -> (junction 14)
    (junction 16) -> (junction 15)
    (junction 17) -> (junction 16)
    (junction 12) -> (junction 18)
  state EastCalc
    entry:
    leftCounter = y-1;
    rightCounter = y-1;
    ULSL = 0;
    ULSR = 0;
    startLeft = true;
    startRight = true;
    state ULSL [parallel]
      settings: executionOrder=2
      (history)
      state ULSL_Calc
      state Hit
      EastCalc.ULSL.ULSL_Calc -> (junction 172) : [leftCounter - 1 >= 0]{leftCounter--;}
      (default) -> EastCalc.ULSL.ULSL_Calc
      (junction 172) -> EastCalc.ULSL.Hit [order 1] : [room[x-1][leftCounter] == 0]
          | /startLeft = false;
      (junction 172) -> EastCalc.ULSL.ULSL_Calc [order 2] : [room[x-1][leftCounter] == 255]
          | /ULSL++;
      EastCalc.ULSL.Hit -> EastCalc.ULSL.ULSL_Calc : [startLeft]
    state ULSR [parallel]
      settings: executionOrder=1
      (history)
      state ULSR_Calc1
      state Hit
      EastCalc.ULSR.ULSR_Calc1 -> (junction 185) : [rightCounter + 1 <= roomSize]{rightCounter++;}
      (default) -> EastCalc.ULSR.ULSR_Calc1
      (junction 185) -> EastCalc.ULSR.Hit [order 1] : [room[x-1][rightCounter] == 0]
          | /startRight = false;
      (junction 185) -> EastCalc.ULSR.ULSR_Calc1 [order 2] : [room[x-1][rightCounter] == 255]
          | /ULSR++;
      EastCalc.ULSR.Hit -> EastCalc.ULSR.ULSR_Calc1 : [startRight]
  state SouthCalc
    entry:
    leftCounter = x-1;
    rightCounter = x-1;
    ULSL = 0;
    ULSR = 0;
    startLeft = true;
    startRight = true;
    state ULSL [parallel]
      settings: executionOrder=2
      (history)
      state ULSL_Calc
      state Hit
      SouthCalc.ULSL.ULSL_Calc -> (junction 226) : [leftCounter + 1 <= roomSize]{leftCounter++;}
      (default) -> SouthCalc.ULSL.ULSL_Calc
      (junction 226) -> SouthCalc.ULSL.Hit [order 1] : [room[leftCounter][y-1] == 0]
          | /startLeft = false;
      (junction 226) -> SouthCalc.ULSL.ULSL_Calc [order 2] : [room[leftCounter][y-1] == 255]
          | /ULSL++;
      SouthCalc.ULSL.Hit -> SouthCalc.ULSL.ULSL_Calc : [startLeft]
    state ULSR [parallel]
      settings: executionOrder=1
      (history)
      state ULSR_Calc
      state Hit
      SouthCalc.ULSR.ULSR_Calc -> (junction 213) : [rightCounter - 1 >= 0]{rightCounter--;}
      (default) -> SouthCalc.ULSR.ULSR_Calc
      (junction 213) -> SouthCalc.ULSR.Hit [order 1] : [room[rightCounter][y - 1] == 0]
          | /startRight = false;
      (junction 213) -> SouthCalc.ULSR.ULSR_Calc [order 2] : [room[rightCounter][y - 1] == 255]
          | /ULSR++;
      SouthCalc.ULSR.Hit -> SouthCalc.ULSR.ULSR_Calc : [startRight]
  (default) -> CalcHeading
  CalcHeading -> WestCalc [order 1] : [(heading == WEST) ...
      | && (hasChanged(heading)...
      | || hasChanged(x))]
      | /readingReady = false;
  CalcHeading -> NorthCalc [order 4] : [(heading == NORTH) ...
      | && (hasChanged(heading)...
      | || hasChanged(y))]
      | /readingReady = false;
  WestCalc -> (junction 154) : [x-1 >= 0]
  (junction 154) -> CalcHeading : [(room[x-1][rightCounter] == 0)...
      |  &&(room[x-1][leftCounter] == 0)]
      | /readingReady = true;
  NorthCalc -> (junction 117) : [y-1 >= 0]
  EastCalc -> (junction 154) : [x-1 >= 0]
  (junction 117) -> CalcHeading : [(room[rightCounter][y-1] == 0)...
      |  &&(room[leftCounter][y-1] == 0)]
      | /readingReady = true;
  SouthCalc -> (junction 117) : [y-1 >= 0]
  CalcHeading -> EastCalc [order 2] : [(heading == EAST) ...
      | && (hasChanged(heading)...
      | || hasChanged(x))]
      | /readingReady = false;
  CalcHeading -> SouthCalc [order 3] : [(heading == SOUTH) ...
      | && (hasChanged(heading)...
      | || hasChanged(y))]
      | /readingReady = false;
  CalcHeading -> CalcHeading [order 5] : [hasChanged(theta)]
  data: ERRVAL input; NORTH input; SOUTH input; EAST input; WEST input; NONE input; room input size=[ROOM_SIDE_SIZE*BLOCK_SIZE/4 ROOM_SIDE_SIZE*BLOCK_SIZE/4]; heading local int16; theta input; Vl input; Vr input; roomSize input; x input; y input; wrongHeading_BOOL output double; ULSL output double; ULSR output double; leftCounter local double; rightCounter local double; startLeft local boolean; startRight local boolean; readingReady output boolean

== matlab function AreaCoverageTestHarness/Robot/DetailedMap/createMap/RoomV1/Room_V1 ==
  data: roomOut output size=[ROOM_SIDE_SIZE*BLOCK_SIZE/4 ROOM_SIDE_SIZE*BLOCK_SIZE/4] [0..255]; ROOM_SIDE_SIZE parameter; BLOCK_SIZE parameter
function roomOut = fcn(ROOM_SIDE_SIZE, BLOCK_SIZE)

persistent flag;
persistent room;
   side_size = ROOM_SIDE_SIZE * (BLOCK_SIZE/4);

if isempty(flag)
    flag = false;
    room = uint8(ones(side_size , side_size)*255);
end

if flag == false
   flag = true;
%     room = uint8(ones(ROOM_SIDE_SIZE , ROOM_SIDE_SIZE)*255);

    %% Draw room Boarders
    for rowNum = 1:(side_size)
        for colNum = 1: side_size
            if (rowNum <= BLOCK_SIZE/4) || (rowNum >= (side_size - BLOCK_SIZE/4))...
                    || (colNum <= BLOCK_SIZE/4) || (colNum >= side_size - BLOCK_SIZE/4)
    %                 || (rowNum == 2) || (rowNum == roomSize - 1)...
    %                 || (colNum == 2) || (colNum == roomSize-1)
                room(rowNum, colNum) = 0;
            end
        end
    end

    %% Draw room Obsticals
    scale = 5;
    %% insert Table
    room((4*scale - scale/2) + 0.5:(4*scale + scale/2) + 0.5, (9*scale - scale/2) + 0.5:(9*scale + scale/2 )+ 0.5) = 0;
    room((6*scale - scale/2) + 0.5:(6*scale + scale/2) + 0.5, (9*scale - scale/2) + 0.5:(9*scale + scale/2 )+ 0.5) = 0;
    room((4*scale - scale/2) + 0.5:(4*scale + scale/2) + 0.5, (11*scale - scale/2) + 0.5:(11*scale + scale/2 )+ 0.5) = 0;
    room((6*scale - scale/2) + 0.5:(6*scale + scale/2) + 0.5, (11*scale - scale/2) + 0.5:(11*scale + scale/2 )+ 0.5) = 0;

    %% insert box

    room((3*scale - scale/2) + 0.5:(4*scale + scale/2) + 0.5, (4*scale - (scale)/2) + 0.5:(5*scale + (scale)/2 )+ 0.5) = 0;

    %% insert soffa
    room((12*scale - scale/2) + 0.5:(14*scale + scale/2) + 0.5, (8*scale + scale/2) + 0.5:(13*scale + scale/2 )+ 0.5) = 0;

    %% insert LeglessTable
    room((7*scale - scale/2) + 0.5:(11*scale + scale/2) + 0.5, (1*scale - scale/2) + 0.5:(4*scale + scale/2 )+ 0.5) = 0;
    
    
    roomOut = room;
else
    roomOut = room;
end

== matlab function AreaCoverageTestHarness/Robot/DetailedMap/createMap/RoomV2/Room_V2 ==
  data: roomOut output size=[ROOM_SIDE_SIZE*BLOCK_SIZE/4 ROOM_SIDE_SIZE*BLOCK_SIZE/4] [0..255]; ROOM_SIDE_SIZE parameter; BLOCK_SIZE parameter
function roomOut = fcn(ROOM_SIDE_SIZE, BLOCK_SIZE)

persistent flag;
persistent room;
   side_size = ROOM_SIDE_SIZE * (BLOCK_SIZE/4);

if isempty(flag)
    flag = false;
    room = uint8(ones(side_size , side_size)*255);
end

if flag == false
   flag = true;
%     room = uint8(ones(ROOM_SIDE_SIZE , ROOM_SIDE_SIZE)*255);

    %% Draw room Boarders
    for rowNum = 1:(side_size)
        for colNum = 1: side_size
            if (rowNum <= BLOCK_SIZE/4) || (rowNum >= (side_size - BLOCK_SIZE/4))...
                    || (colNum <= BLOCK_SIZE/4) || (colNum >= side_size - BLOCK_SIZE/4)
    %                 || (rowNum == 2) || (rowNum == roomSize - 1)...
    %                 || (colNum == 2) || (colNum == roomSize-1)
                room(rowNum, colNum) = 0;
            end
        end
    end

    %% Draw room Obsticals
    scale = 5;
    %% insert Table
    room((14*scale - scale/2) + 0.5:(19*scale + scale/2) + 0.5, (4*scale - scale/4) + 0.5:(4*scale + scale/4 )+ 0.5) = 0;
    room((14*scale - scale/2) + 0.5:(19*scale + scale/2) + 0.5, (6*scale - scale/4) + 0.5:(6*scale + scale/4 )+ 0.5) = 0;
    room((14*scale - scale/2) + 0.5:(19*scale + scale/2) + 0.5, (8*scale - scale/4) + 0.5:(8*scale + scale/4 )+ 0.5) = 0;
    room((14*scale - scale/2) + 0.5:(19*scale + scale/2) + 0.5, (10*scale - scale/4) + 0.5:(10*scale + scale/4 )+ 0.5) = 0;
    room((14*scale - scale/2) + 0.5:(19*scale + scale/2) + 0.5, (12*scale - scale/4) + 0.5:(12*scale + scale/4 )+ 0.5) = 0;
    room((18.5*scale - scale/2) + 0.5:(19*scale + scale/2) + 0.5, (14*scale - scale/2) + 0.5:(14*scale + scale/2 )+ 0.5) = 0;

    %% insert box

    room((10*scale - scale/2) + 0.5:(19*scale + scale/2) + 0.5, (1*scale - (scale)/2) + 0.5:(3*scale + (scale)/2 )+ 0.5) = 0;

    %% insert soffa
    room((1*scale - scale/2) + 0.5:(4*scale + scale/2) + 0.5, (8*scale - (scale)/2) + 0.5:(19*scale + (scale)/2 )+ 0.5) = 0;

    %% insert LeglessTable
    room((7*scale - scale/2) + 0.5:(11*scale + scale/2) + 0.5, (1*scale - scale/2) + 0.5:(4*scale + scale/2 )+ 0.5) = 0;
    
    room((4*scale - scale/2) + 0.5:(19*scale + scale/2) + 0.5, (16*scale - scale/2) + 0.5:(19*scale + scale/2 )+ 0.5) = 0;

    
    roomOut = room;
else
    roomOut = room;
end
